simulink model "Subsystem"  (R2020b)
settings: Solver=FixedStepDiscrete  StartTime=0.0  StopTime=10.0  FixedStep=1  RelTol=1e-3
model workspace (MAT data in the model file):
  K1 = 1
  K2 = 2
  K3 = -3
  K4 = -4
  K5 = 5
settings Model: Creator=user  LastModifiedBy=user
settings DataIOCC: SaveOutput=off  SaveTime=off

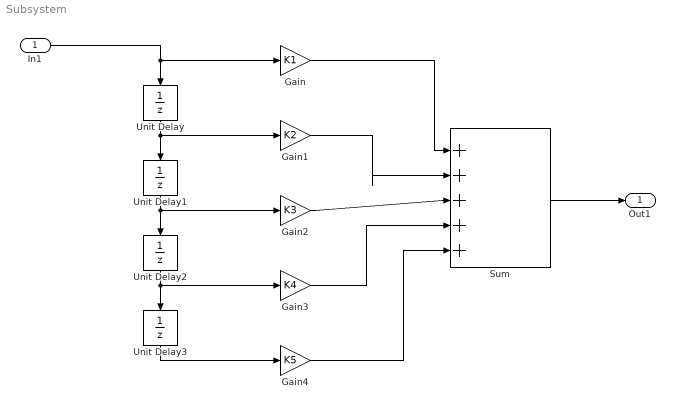
== system Subsystem ==
  In1 : Inport  OutDataTypeStr=double  PortDimensions=1  SampleTime=0
  Gain : Gain  Gain=K1
  Gain1 : Gain  Gain=K2
  Gain2 : Gain  Gain=K3
  Gain3 : Gain  Gain=K4
  Gain4 : Gain  Gain=K5
  Sum : Sum  Inputs=+|++++
  Unit Delay{,1..3} (4 alike) : UnitDelay  SampleTime=-1  HasFrameUpgradeWarning=on
  Out1 : Outport  OutDataTypeStr=double  PortDimensions=1  SampleTime=0
  wires:
  Gain2/1 -> Sum/3
  Gain3/1 -> Sum/4
  Unit Delay2/1 -> Unit Delay3/1, Gain3/1
  Gain/1 -> Sum/1
  Unit Delay/1 -> Unit Delay1/1, Gain1/1
  Unit Delay3/1 -> Gain4/1
  Unit Delay1/1 -> Unit Delay2/1, Gain2/1
  Gain4/1 -> Sum/5
  Gain1/1 -> Sum/2
  In1/1 -> Gain/1, Unit Delay/1
  Sum/1 -> Out1/1
